simulink model "PSD"  (R2024b)
settings: Solver=VariableStepAuto  StartTime=0.0  StopTime=10.0  RelTol=1e-3
values from neighbouring files (symbols this model uses):
  D = K * (Td / Tvz)    [PID2PSDSquares.m]    (also in PID2PSDTrapezoids.m = Kp * (Td / Tvz))
  P = [1]    [DeadBeat.m]    (also in DeadBeatRestrained.m; PID2PSDSquares.m = Kp * (1 + (Td / Tvz)); PID2PSDTrapezoids.m = Kp * (1 + (Tvz / (2 * Ti)) + (Td / Tvz)); PolesPlacement.m = double([1; P(:)])')
  S = - K * (1 + 2 * (Td / Tvz) - (Tvz / Ti))    [PID2PSDSquares.m]    (also in PID2PSDTrapezoids.m = - Kp * (1 + 2 * (Td / Tvz) - (Tvz / (2 * Ti))))
undefined symbols (not defined in the file or in its folder): Tvz
settings Model: Creator=lukiq  LastModifiedBy=lukiq

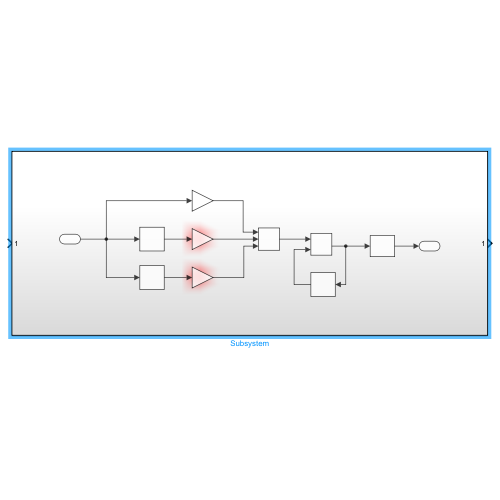
[thumbnail: Simulink's stored preview of the top-level diagram]
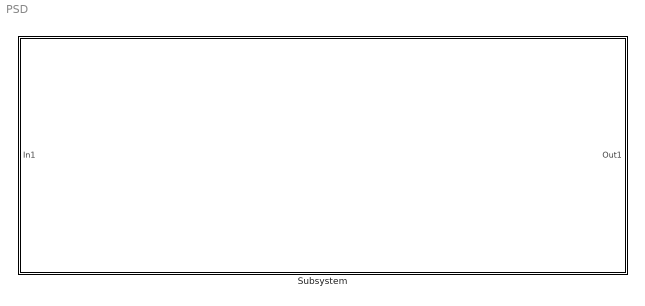
== system PSD ==
  Subsystem : Subsystem

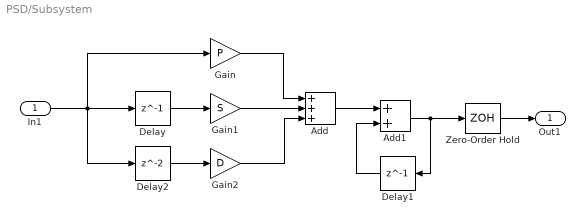
== system PSD/Subsystem ==
  In1 : Inport
  Add : Sum  Inputs=+++
  Add1 : Sum
  Delay : Delay  DelayLength=1  SampleTime=Tvz
  Delay1 : Delay  DelayLength=1  SampleTime=Tvz
  Delay2 : Delay  SampleTime=Tvz
  Gain : Gain  Gain=P
  Gain1 : Gain  Gain=S
  Gain2 : Gain  Gain=D
  Zero-Order Hold : ZeroOrderHold  SampleTime=Tvz
  Out1 : Outport
  wires:
  Gain2/1 -> Add/3
  In1/1 -> Delay2/1, Delay/1, Gain/1
  Delay1/1 -> Add1/2
  Zero-Order Hold/1 -> Out1/1
  Add1/1 -> Delay1/1, Zero-Order Hold/1
  Delay2/1 -> Gain2/1
  Gain/1 -> Add/1
  Delay/1 -> Gain1/1
  Gain1/1 -> Add/2
  Add/1 -> Add1/1
